simulink model "VirtualDAQ2_issue"  (R2021b)
settings: Solver=VariableStepAuto  StartTime=0.0  StopTime=inf  MaxStep=0.001  RelTol=1e-3
libraries: fl_lib x5, nesl_utility x3, simulink x2
(part 2 of 2)

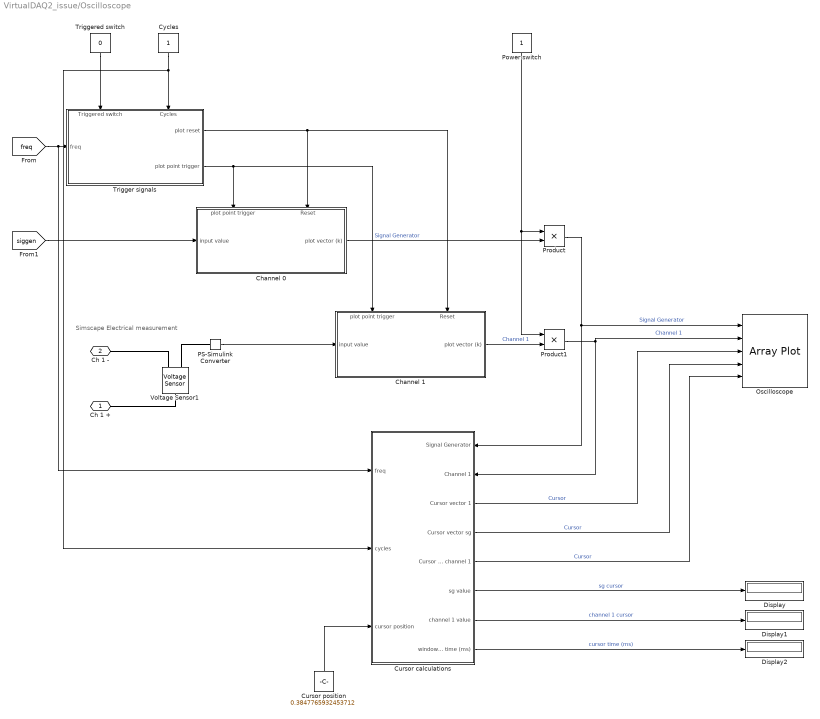
== system VirtualDAQ2_issue/Oscilloscope ==
  note: Simscape Electrical measurement
  Channel 0 : Subsystem
      settings: PortSchema="{\"entries\":[{\"content\":{\"sides\":[{\"content\":{\"connectorIds\":[\"In1\"]},\"type\":\"ConnectorPlacement.EquallySpacedRectSide\",\"uuid\":\"56eea059-d5e9-4d95-b7d9-83a317b3103e\"},{\"content\":{\"connectorIds\":[\"Out1\"],\"side\":\"RIGHT\"},\"type\":\"ConnectorPlacement.EquallySpacedRectSide\",\"uuid\":\"fd8b8cd5-6def-4d8f-87ca-646372cc7fbe\"},{\"content\":{\"connectorIds\":[\"In2\",\"In3\"],\"side\":\"TOP\"},\"type\":\"ConnectorPlacement.EquallySpacedRectSide\",\"uuid\":\"3d9c38ee-b24b-466c-a7ac-a6d8a7456d51\"},{\"content\":{\"connectorIds\":[],\"side\":\"BOTTOM\"},\"type\":\"ConnectorPlacement.EquallySpacedRectSide\",\"uuid\":\"336136fa-2514-49ab-9e17-88caaca7366c\"}]},\"type\":\"ConnectorPlacement.EquallySpacedConnector\",\"uuid\":\"1d9824a8-6efd-49ff-b082-cf2ede19b4fd\"}],\"packageUris\":[\"http://schema.mathworks.com/mf0/Connector/R2020b\"],\"version\":\"1.0\"}"
  Channel 1 : Subsystem
      settings: PortSchema="{\"entries\":[{\"content\":{\"sides\":[{\"content\":{\"connectorIds\":[\"In1\"]},\"type\":\"ConnectorPlacement.EquallySpacedRectSide\",\"uuid\":\"56eea059-d5e9-4d95-b7d9-83a317b3103e\"},{\"content\":{\"connectorIds\":[\"Out1\"],\"side\":\"RIGHT\"},\"type\":\"ConnectorPlacement.EquallySpacedRectSide\",\"uuid\":\"fd8b8cd5-6def-4d8f-87ca-646372cc7fbe\"},{\"content\":{\"connectorIds\":[\"In2\",\"In3\"],\"side\":\"TOP\"},\"type\":\"ConnectorPlacement.EquallySpacedRectSide\",\"uuid\":\"3d9c38ee-b24b-466c-a7ac-a6d8a7456d51\"},{\"content\":{\"connectorIds\":[],\"side\":\"BOTTOM\"},\"type\":\"ConnectorPlacement.EquallySpacedRectSide\",\"uuid\":\"336136fa-2514-49ab-9e17-88caaca7366c\"}]},\"type\":\"ConnectorPlacement.EquallySpacedConnector\",\"uuid\":\"1d9824a8-6efd-49ff-b082-cf2ede19b4fd\"}],\"packageUris\":[\"http://schema.mathworks.com/mf0/Connector/R2020b\"],\"version\":\"1.0\"}"
  Cursor calculations : Subsystem
      settings: PortSchema="{\"entries\":[{\"content\":{\"sides\":[{\"content\":{\"connectorIds\":[\"In1\",\"In2\",\"In3\"]},\"type\":\"ConnectorPlacement.EquallySpacedRectSide\",\"uuid\":\"1c989ad6-e53e-4c35-b3b5-c49236b4c481\"},{\"content\":{\"connectorIds\":[\"In4\",\"In5\",\"Out1\",\"Out2\",\"Out3\",\"Out4\",\"Out5\",\"Out6\"],\"side\":\"RIGHT\"},\"type\":\"ConnectorPlacement.EquallySpacedRectSide\",\"uuid\":\"f7f12d6e-f108-4402-9333-d7b82b87f80e\"},{\"content\":{\"connectorIds\":[],\"side\":\"TOP\"},\"type\":\"ConnectorPlacement.EquallySpacedRectSide\",\"uuid\":\"66ce7c3f-d403-4718-8f25-8060696ddae9\"}]},\"type\":\"ConnectorPlacement.EquallySpacedConnector\",\"uuid\":\"8d64b060-7a87-4186-b73c-eb27c1ca19d1\"}],\"packageUris\":[\"http://schema.mathworks.com/mf0/Connector/R2020b\"],\"version\":\"1.0\"}"
  Cursor position : Constant  Value=0.3847765932453712
  Cycles : Constant
  Display : Display
  Display1 : Display
  Display2 : Display
  Oscilloscope : ArrayPlot  NumInputPorts=5  WindowPosition=[1282.000000,42.000000,1279.000000,1369.000000,]  Visible=on  PlotType=Line  AxesScaling=Manual  YLimits=[-5.1,5.1]  ShowLegend=on
  PS-Simulink Converter : nesl_utility/PS-Simulink Converter  PhysicalDomain=network_engine_domain  SubClassName=ps_output  LeftPortType=input  RightPortType=output  PseudoPeriodic=off  Frequencies=[]  Unit=inherit  AffineConversion=off
      settings: SourceProductBaseCode=PW,SS
  Power switch : Constant
  Product : Product
  Product1 : Product
  Trigger signals : Subsystem
      settings: PortSchema="{\"entries\":[{\"content\":{\"sides\":[{\"content\":{\"connectorIds\":[\"In1\"]},\"type\":\"ConnectorPlacement.EquallySpacedRectSide\",\"uuid\":\"b92255b7-066e-487b-9e0c-e19692fc940f\"},{\"content\":{\"connectorIds\":[\"Out1\",\"Out2\"],\"side\":\"RIGHT\"},\"type\":\"ConnectorPlacement.EquallySpacedRectSide\",\"uuid\":\"cb964d42-f40b-466c-b45b-853437324272\"},{\"content\":{\"connectorIds\":[\"In2\",\"In3\"],\"side\":\"TOP\"},\"type\":\"ConnectorPlacement.EquallySpacedRectSide\",\"uuid\":\"e1027385-b295-47a3-ae7d-2e3bb07fa1de\"}]},\"type\":\"ConnectorPlacement.EquallySpacedConnector\",\"uuid\":\"1db11e79-2cf0-4841-86d9-651820ebc8ee\"}],\"packageUris\":[\"http://schema.mathworks.com/mf0/Connector/R2020b\"],\"version\":\"1.0\"}"
  Triggered switch : Constant  Value=0
  Voltage Sensor1 : fl_lib/Electrical/Electrical Sensors/Voltage Sensor
  Ch 1 + : PMIOPort  Side=Right
  Ch 1 - : PMIOPort  Port=2  Side=Right
  wires:
  PS-Simulink Converter/1 -> Channel 1/1(input value)
  Trigger signals/1("plot reset ") -> Channel 0/3(Reset), Channel 1/3(Reset)
  Product1/1 -> Cursor calculations/5(Channel 1), Oscilloscope/2  "Channel 1"
  Trigger signals/2(plot point trigger) -> Channel 0/2(plot point trigger), Channel 1/2(plot point trigger)
  [freq] -> Cursor calculations/1(freq), Trigger signals/1(freq)
  Product/1 -> Cursor calculations/4(Signal Generator), Oscilloscope/1  "Signal Generator"
  [siggen] -> Channel 0/1(input value)
  Power switch/1 -> Product1/1, Product/1
  Channel 0/1(plot vector (k)) -> Product/2  "Signal Generator"
  Channel 1/1(plot vector (k)) -> Product1/2  "Channel 1"
  Triggered switch/1 -> Trigger signals/2(Triggered switch)
  Cycles/1 -> Trigger signals/3(Cycles), Cursor calculations/2(cycles)
  Cursor position/1 -> Cursor calculations/3(cursor position)
  Cursor calculations/1(Cursor vector 1) -> Oscilloscope/3  "Cursor"
  Cursor calculations/4(sg value) -> Display/1  "sg cursor"
  Cursor calculations/5(channel 1 value) -> Display1/1  "channel 1 cursor"
  Cursor calculations/3(Cursor vector channel 1) -> Oscilloscope/5  "Cursor"
  Cursor calculations/6(window time (ms)) -> Display2/1  "cursor time (ms)"
  Cursor calculations/2(Cursor vector sg) -> Oscilloscope/4  "Cursor"
  connections:
  Voltage Sensor1/RConn2 -- Ch 1 -/RConn1
  Voltage Sensor1/RConn1 -- PS-Simulink Converter/LConn1
  Voltage Sensor1/LConn1 -- Ch 1 +/RConn1

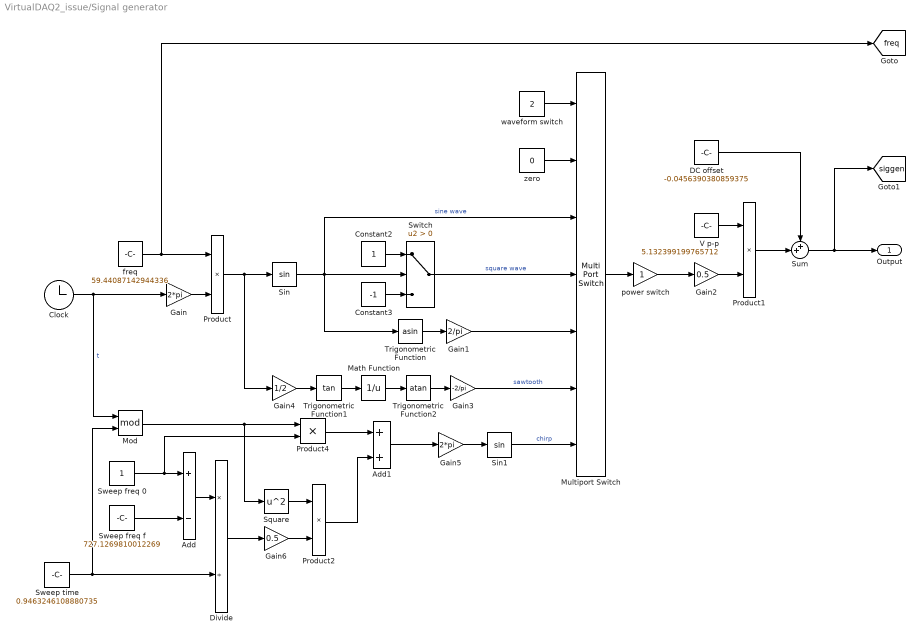
== system VirtualDAQ2_issue/Signal generator ==
  Add : Sum  Inputs=+-
  Add1 : Sum
  Clock : Clock
  Constant2 : Constant  SampleTime=0
  Constant3 : Constant  Value=-1  SampleTime=0
  DC offset : Constant  Value=-0.0456390380859375
  Divide : Product  Inputs=*/
  Gain : Gain  Gain=2*pi
  Gain1 : Gain  Gain=2/pi
  Gain2 : Gain  Gain=0.5
  Gain3 : Gain  Gain=-2/pi
  Gain4 : Gain  Gain=1/2
  Gain5 : Gain  Gain=2*pi
  Gain6 : Gain  Gain=0.5
  Math Function : Math  Operator=reciprocal  SaturateOnIntegerOverflow=on
  Mod : Math  Operator=mod  SaturateOnIntegerOverflow=on
  Multiport Switch : MultiPortSwitch  DataPortOrder=Zero-based contiguous  Inputs=6  DiagnosticForDefault=None  zeroidx=on
  Product{,1..2,4} (4 alike) : Product
  Sin : Trigonometry
  Sin1 : Trigonometry
  Square : Math  Operator=square  SaturateOnIntegerOverflow=on
  Sum : Sum  Inputs=++|
  Sweep freq 0 : Constant
  Sweep freq f : Constant  Value=727.1269810012269
  Sweep time : Constant  Value=0.9463246108880735
  Switch : Switch  Criteria=u2 > Threshold
  Trigonometric Function : Trigonometry  Operator=asin
  Trigonometric Function1 : Trigonometry  Operator=tan
  Trigonometric Function2 : Trigonometry  Operator=atan
  V p-p : Constant  Value=5.132399199765712  SampleTime=-1
  freq : Constant  Value=59.44087142944336  SampleTime=0
  power switch : Gain
  waveform switch : Constant  Value=2  SampleTime=0
  zero : Constant  Value=0  SampleTime=0
  Output : Outport
  tag scope: freq=global, siggen=global
  wires:
  Sin/1 -> Trigonometric Function/1, Multiport Switch/3, Switch/2  "sine wave"
  freq/1 -> [freq], Product/1
  Clock/1 -> Gain/1, Mod/1  "t"
  power switch/1 -> Gain2/1
  zero/1 -> Multiport Switch/2
  Sin1/1 -> Multiport Switch/7  "chirp"
  Trigonometric Function/1 -> Gain1/1
  Constant2/1 -> Switch/1
  Constant3/1 -> Switch/3
  Gain2/1 -> Product1/2
  Product/1 -> Sin/1, Gain4/1
  Gain1/1 -> Multiport Switch/5
  waveform switch/1 -> Multiport Switch/1
  Math Function/1 -> Trigonometric Function2/1
  Trigonometric Function1/1 -> Math Function/1
  Trigonometric Function2/1 -> Gain3/1
  Gain4/1 -> Trigonometric Function1/1
  Multiport Switch/1 -> power switch/1
  Gain3/1 -> Multiport Switch/6  "sawtooth"
  V p-p/1 -> Product1/1
  Product1/1 -> Sum/2
  DC offset/1 -> Sum/1
  Switch/1 -> Multiport Switch/4  "square wave"
  Sum/1 -> [siggen], Output/1
  Sweep freq 0/1 -> Product4/2, Add/1
  Sweep freq f/1 -> Add/2
  Add/1 -> Divide/1
  Sweep time/1 -> Mod/2, Divide/2
  Gain5/1 -> Sin1/1
  Add1/1 -> Gain5/1
  Divide/1 -> Gain6/1
  Gain/1 -> Product/2
  Product4/1 -> Add1/1
  Square/1 -> Product2/1
  Gain6/1 -> Product2/2
  Product2/1 -> Add1/2
  Mod/1 -> Product4/1, Square/1

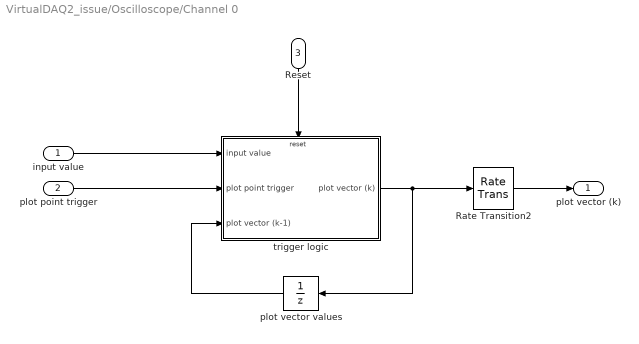
== system VirtualDAQ2_issue/Oscilloscope/Channel 0 ==
  input value : Inport
  plot point trigger : Inport  Port=2
  Reset : Inport  Port=3
  Rate Transition2 : RateTransition  OutPortSampleTime=1/refreshRate
  plot vector values : UnitDelay  InitialCondition=zeros(Np,1)  SampleTime=-1  HasFrameUpgradeWarning=on
  trigger logic : Subsystem  TreatAsAtomicUnit=on
  plot vector (k) : Outport
  wires:
  plot vector values/1 -> trigger logic/3(plot vector (k-1))
  plot point trigger/1 -> trigger logic/2(plot point trigger)
  trigger logic/1(plot vector (k)) -> Rate Transition2/1, plot vector values/1
  Reset/1 -> trigger logic/Reset
  input value/1 -> trigger logic/1(input value)
  Rate Transition2/1 -> plot vector (k)/1

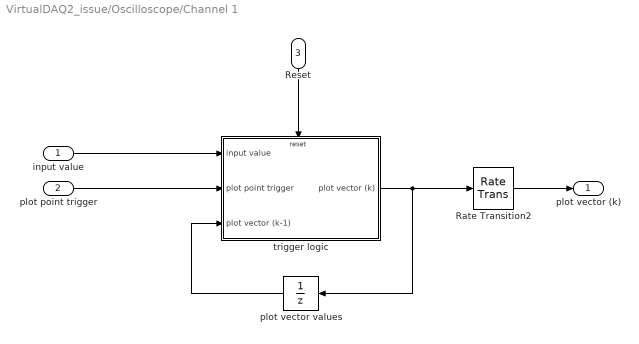
== system VirtualDAQ2_issue/Oscilloscope/Channel 1 ==
  input value : Inport
  plot point trigger : Inport  Port=2
  Reset : Inport  Port=3
  Rate Transition2 : RateTransition  OutPortSampleTime=1/refreshRate
  plot vector values : UnitDelay  InitialCondition=zeros(Np,1)  SampleTime=-1  HasFrameUpgradeWarning=on
  trigger logic : Subsystem  TreatAsAtomicUnit=on
  plot vector (k) : Outport
  wires:
  plot vector values/1 -> trigger logic/3(plot vector (k-1))
  plot point trigger/1 -> trigger logic/2(plot point trigger)
  trigger logic/1(plot vector (k)) -> Rate Transition2/1, plot vector values/1
  Reset/1 -> trigger logic/Reset
  input value/1 -> trigger logic/1(input value)
  Rate Transition2/1 -> plot vector (k)/1

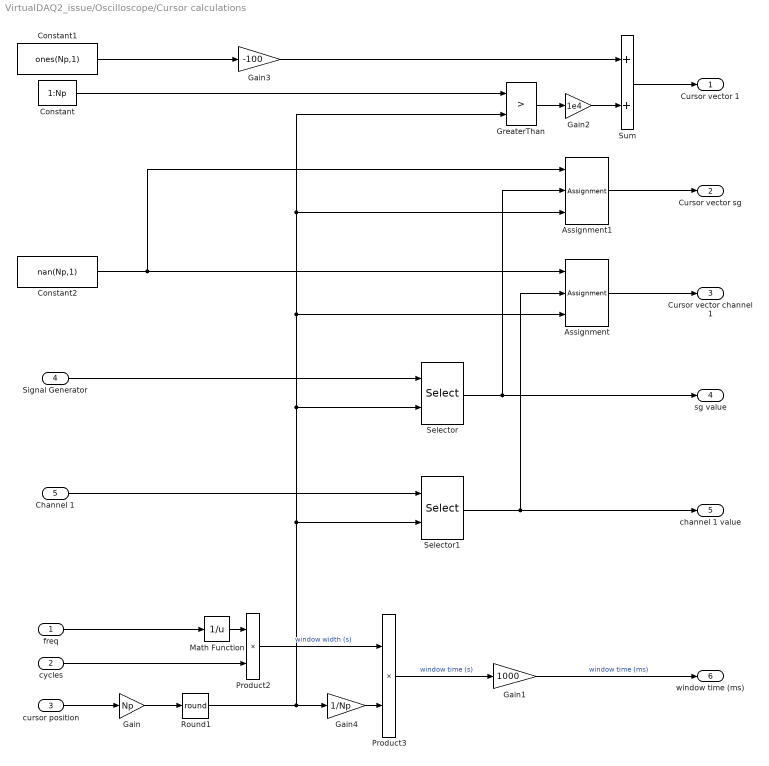
== system VirtualDAQ2_issue/Oscilloscope/Cursor calculations ==
  freq : Inport
  cycles : Inport  Port=2
  cursor position : Inport  Port=3
  Signal Generator : Inport  Port=4
  Channel 1 : Inport  Port=5
  Assignment : Assignment  DiagnosticForDimensions=Warning  IndexOptions=Index vector (port)  Indices=1  OutputSizes=1
  Assignment1 : Assignment  DiagnosticForDimensions=Warning  IndexOptions=Index vector (port)  Indices=1  OutputSizes=1
  Constant : Constant  Value=1:Np
  Constant1 : Constant  Value=ones(Np,1)
  Constant2 : Constant  Value=nan(Np,1)
  Gain : Gain  Gain=Np
  Gain1 : Gain  Gain=1000
  Gain2 : Gain  Gain=1e4
  Gain3 : Gain  Gain=-100
  Gain4 : Gain  Gain=1/Np
  GreaterThan : RelationalOperator  Operator=>  OutDataTypeStr=boolean  RndMeth=Simplest
  Math Function : Math  Operator=reciprocal  SaturateOnIntegerOverflow=on
  Product2 : Product
  Product3 : Product
  Round1 : Rounding  Operator=round
  Selector : Selector  InputPortWidth=Np  IndexOptions=Index vector (port)  Indices=[1 3]  OutputSizes=1
  Selector1 : Selector  InputPortWidth=Np  IndexOptions=Index vector (port)  Indices=[1 3]  OutputSizes=1
  Sum : Sum
  Cursor vector 1 : Outport
  Cursor vector sg : Outport  Port=2
  Cursor vector channel 1 : Outport  Port=3
  sg value : Outport  Port=4
  channel 1 value : Outport  Port=5
  window time (ms) : Outport  Port=6
  wires:
  Math Function/1 -> Product2/1
  cursor position/1 -> Gain/1
  Constant/1 -> GreaterThan/1
  Product2/1 -> Product3/1  "window width (s)"
  cycles/1 -> Product2/2
  freq/1 -> Math Function/1
  Product3/1 -> Gain1/1  "window time (s)"
  Gain1/1 -> window time (ms)/1  "window time (ms)"
  GreaterThan/1 -> Gain2/1
  Sum/1 -> Cursor vector 1/1
  Gain2/1 -> Sum/2
  Signal Generator/1 -> Selector/1
  Selector1/1 -> Assignment/2, channel 1 value/1
  Constant1/1 -> Gain3/1
  Gain3/1 -> Sum/1
  Gain/1 -> Round1/1
  Gain4/1 -> Product3/2
  Channel 1/1 -> Selector1/1
  Assignment/1 -> Cursor vector channel 1/1
  Selector/1 -> Assignment1/2, sg value/1
  Assignment1/1 -> Cursor vector sg/1
  Round1/1 -> Selector/2, Assignment1/3, GreaterThan/2, Assignment/3, Selector1/2, Gain4/1
  Constant2/1 -> Assignment1/1, Assignment/1

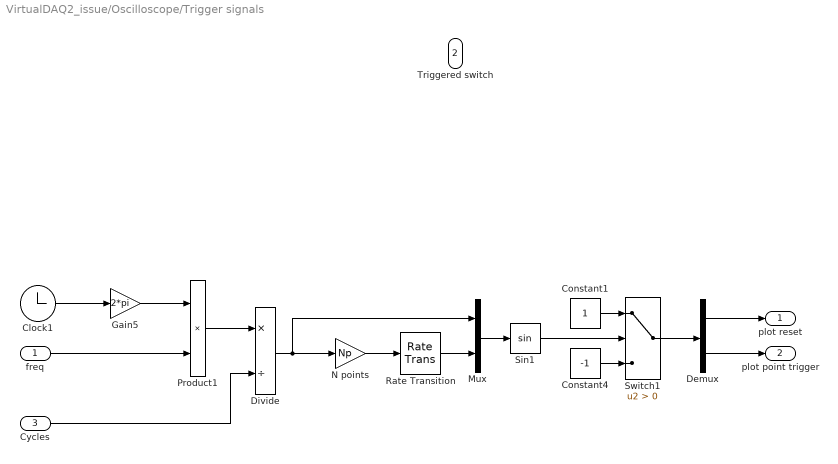
== system VirtualDAQ2_issue/Oscilloscope/Trigger signals ==
  freq : Inport
  Triggered switch : Inport  Port=2
  Cycles : Inport  Port=3
  Clock1 : Clock
  Constant1 : Constant  SampleTime=0
  Constant4 : Constant  Value=-1  SampleTime=0
  Demux : Demux  Outputs=2
  Divide : Product  Inputs=*/
  Gain5 : Gain  Gain=2*pi
  Mux : Mux  Inputs=2
  N points : Gain  Gain=Np
  Product1 : Product
  Rate Transition : RateTransition  OutPortSampleTime=plot_dt
  Sin1 : Trigonometry
  Switch1 : Switch  Criteria=u2 > Threshold
  "plot reset " : Outport
  plot point trigger : Outport  Port=2
  wires:
  Gain5/1 -> Product1/1
  Constant4/1 -> Switch1/3
  Clock1/1 -> Gain5/1
  Sin1/1 -> Switch1/2
  Constant1/1 -> Switch1/1
  freq/1 -> Product1/2
  Product1/1 -> Divide/1
  Divide/1 -> Mux/1, N points/1
  N points/1 -> Rate Transition/1
  Mux/1 -> Sin1/1
  Switch1/1 -> Demux/1
  Demux/2 -> plot point trigger/1
  Demux/1 -> "plot reset "/1
  Rate Transition/1 -> Mux/2
  Cycles/1 -> Divide/2

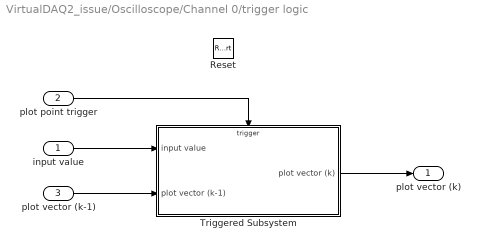
== system VirtualDAQ2_issue/Oscilloscope/Channel 0/trigger logic ==
  input value : Inport
  plot point trigger : Inport  Port=2
  plot vector (k-1) : Inport  Port=3
  Reset : ResetPort  DisableCoverage=on
  Triggered Subsystem : Subsystem  TreatAsAtomicUnit=on
  plot vector (k) : Outport
  wires:
  plot point trigger/1 -> Triggered Subsystem/Trigger
  input value/1 -> Triggered Subsystem/1(input value)
  Triggered Subsystem/1(plot vector (k)) -> plot vector (k)/1
  plot vector (k-1)/1 -> Triggered Subsystem/2(plot vector (k-1))

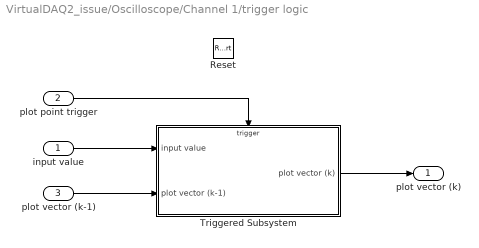
== system VirtualDAQ2_issue/Oscilloscope/Channel 1/trigger logic ==
  input value : Inport
  plot point trigger : Inport  Port=2
  plot vector (k-1) : Inport  Port=3
  Reset : ResetPort  DisableCoverage=on
  Triggered Subsystem : Subsystem  TreatAsAtomicUnit=on
  plot vector (k) : Outport
  wires:
  plot point trigger/1 -> Triggered Subsystem/Trigger
  input value/1 -> Triggered Subsystem/1(input value)
  Triggered Subsystem/1(plot vector (k)) -> plot vector (k)/1
  plot vector (k-1)/1 -> Triggered Subsystem/2(plot vector (k-1))

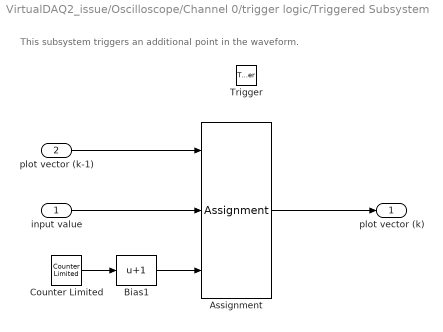
== system VirtualDAQ2_issue/Oscilloscope/Channel 0/trigger logic/Triggered Subsystem ==
  note: This subsystem triggers an additional point in the waveform.
  input value : Inport
  plot vector (k-1) : Inport  Port=2
  Trigger : TriggerPort  VariantControl=(inherit)
  Assignment : Assignment  DiagnosticForDimensions=Warning  IndexOptions=Index vector (port)  Indices=1  OutputSizes=1
  Bias1 : Bias  Bias=1
  Counter Limited : simulink/Sources/Counter Limited  uplimit=Np-1  tsamp=-1
  plot vector (k) : Outport
  wires:
  Assignment/1 -> plot vector (k)/1
  input value/1 -> Assignment/2
  Counter Limited/1 -> Bias1/1
  Bias1/1 -> Assignment/3
  plot vector (k-1)/1 -> Assignment/1

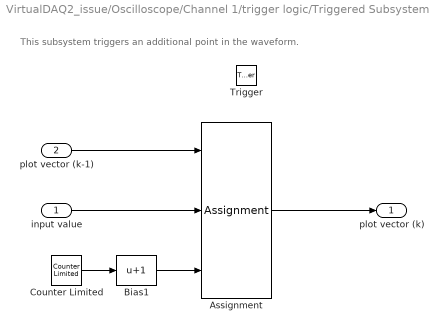
== system VirtualDAQ2_issue/Oscilloscope/Channel 1/trigger logic/Triggered Subsystem ==
  note: This subsystem triggers an additional point in the waveform.
  input value : Inport
  plot vector (k-1) : Inport  Port=2
  Trigger : TriggerPort  VariantControl=(inherit)
  Assignment : Assignment  DiagnosticForDimensions=Warning  IndexOptions=Index vector (port)  Indices=1  OutputSizes=1
  Bias1 : Bias  Bias=1
  Counter Limited : simulink/Sources/Counter Limited  uplimit=Np-1  tsamp=-1
  plot vector (k) : Outport
  wires:
  Assignment/1 -> plot vector (k)/1
  input value/1 -> Assignment/2
  Counter Limited/1 -> Bias1/1
  Bias1/1 -> Assignment/3
  plot vector (k-1)/1 -> Assignment/1
